simulink model "Copy_of_InctanceConfig"  (R2023a)
settings: Solver=VariableStepAuto  StartTime=0.0  StopTime=10.0  RelTol=1e-3
settings Model: Creator=Franz  LastModifiedBy=Franz

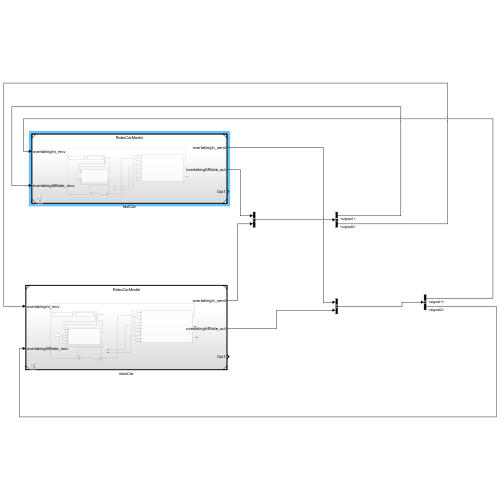
[thumbnail: Simulink's stored preview of the top-level diagram]
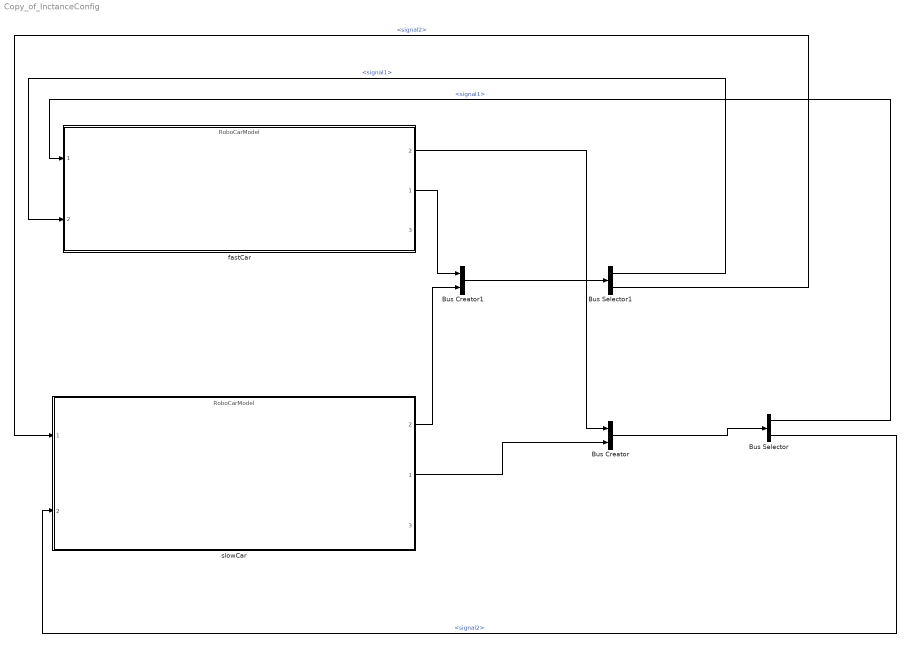
== system Copy_of_InctanceConfig ==
  Bus Creator : BusCreator  Inputs=2
  Bus Creator1 : BusCreator  Inputs=2
  Bus Selector : BusSelector  OutputSignals=signal1,signal2
  Bus Selector1 : BusSelector  OutputSignals=signal1,signal2
  fastCar : ModelReference  ModelNameDialog=RoboCarModel.slx  SimulationMode=Normal  ModelReferenceVersion=1.75
      settings: PortSchema="{\"entries\":[{\"content\":{\"sides\":[{\"content\":{\"connectorIds\":[\"In1\",\"In2\"]},\"type\":\"ConnectorPlacement.EquallySpacedRectSide\",\"uuid\":\"95733cf0-032d-453a-9995-7e8d3e1a24c3\"},{\"content\":{\"connectorIds\":[\"Out2\",\"Out1\",\"Out3\"],\"side\":\"RIGHT\"},\"type\":\"ConnectorPlacement.EquallySpacedRectSide\",\"uuid\":\"8d40af39-e74b-4bad-b693-9b5567a60d93\"},{\"content\":{\"side\":\"TOP\"},\"type\":\"ConnectorPlacement.EquallySpacedRectSide\",\"uuid\":\"43bbd94f-fc32-448c-b6cd-ad2d068142f7\"}]},\"type\":\"ConnectorPlacement.EquallySpacedConnector\",\"uuid\":\"f2b8ce5d-c214-4fd8-985d-570b817192f6\"}],\"packageUris\":[\"http://schema.mathworks.com/mf0/Connector/R2020b\"],\"version\":\"1.0\"}"
  slowCar : ModelReference  ModelNameDialog=RoboCarModel.slx  SimulationMode=Normal  ModelReferenceVersion=1.75
      settings: PortSchema="{\"entries\":[{\"content\":{\"sides\":[{\"content\":{\"connectorIds\":[\"In1\",\"In2\"]},\"type\":\"ConnectorPlacement.EquallySpacedRectSide\",\"uuid\":\"95733cf0-032d-453a-9995-7e8d3e1a24c3\"},{\"content\":{\"connectorIds\":[\"Out2\",\"Out1\",\"Out3\"],\"side\":\"RIGHT\"},\"type\":\"ConnectorPlacement.EquallySpacedRectSide\",\"uuid\":\"8d40af39-e74b-4bad-b693-9b5567a60d93\"},{\"content\":{\"side\":\"TOP\"},\"type\":\"ConnectorPlacement.EquallySpacedRectSide\",\"uuid\":\"43bbd94f-fc32-448c-b6cd-ad2d068142f7\"}]},\"type\":\"ConnectorPlacement.EquallySpacedConnector\",\"uuid\":\"f2b8ce5d-c214-4fd8-985d-570b817192f6\"}],\"packageUris\":[\"http://schema.mathworks.com/mf0/Connector/R2020b\"],\"version\":\"1.0\"}"
  wires:
  Bus Creator/1 -> Bus Selector/1
  fastCar/2 -> Bus Creator/1
  slowCar/1 -> Bus Creator/2
  Bus Selector/1 -> fastCar/1  "<signal1>"
  Bus Selector/2 -> slowCar/2  "<signal2>"
  fastCar/1 -> Bus Creator1/1
  slowCar/2 -> Bus Creator1/2
  Bus Selector1/1 -> fastCar/2  "<signal1>"
  Bus Selector1/2 -> slowCar/1  "<signal2>"
  Bus Creator1/1 -> Bus Selector1/1
